simulink model "ProgettoControlli2_Simulink"  (R2025b)
settings: Solver=VariableStepAuto  StartTime=0.0  StopTime=240  RelTol=1e-3
values from neighbouring files (symbols this model uses):
  beta = 0.08    [progetto.m]    (also in progetto_alternativo.m)
  c = 6.2    [progetto.m]    (also in progetto_alternativo.m)
  Cth = 25.1 * 10^(-3)    (= 0.0251)    [progetto.m]    (also in progetto_alternativo.m)
  dlmax = l/100 * 4    (= 0.006)    [progetto.m]    (also in progetto_alternativo.m)
  g = 9.80665    [progetto.m]    (also in progetto_alternativo.m)
  h = 6.55    [progetto.m]    (also in progetto_alternativo.m)
  J = 2 * 10^(-4)    (= 0.0002)    [progetto.m]    (also in progetto_alternativo.m)
  K_max = 3.92 * 10^3    (= 3920)    [progetto.m]    (also in progetto_alternativo.m)
  m = 0.04    [progetto.m]    (also in progetto_alternativo.m)
  r1 = 0.0045    [progetto.m]    (also in progetto_alternativo.m)
  r2 = 0.045    [progetto.m]    (also in progetto_alternativo.m)
  Re = 4.8    [progetto.m]    (also in progetto_alternativo.m)
  Rth = 16.7    [progetto.m]    (also in progetto_alternativo.m)
  S = pi*d*l    (= 9.42477796077e-05)    [progetto.m]    (also in progetto_alternativo.m)
  Tamb = celsiusToKelvin(24)    [progetto.m]    (also in progetto_alternativo.m)
  Tavg = celsiusToKelvin(70)    [progetto.m]    (also in progetto_alternativo.m)
  Tdiff = 20    [progetto.m]    (also in progetto_alternativo.m)
  Tp = celsiusToKelvin(15)    [progetto.m]    (also in progetto_alternativo.m)
settings Model: Creator=nic  LastModifiedBy=nic

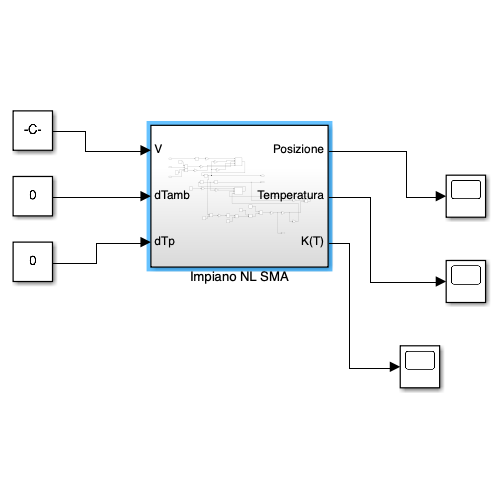
[thumbnail: Simulink's stored preview of the top-level diagram]
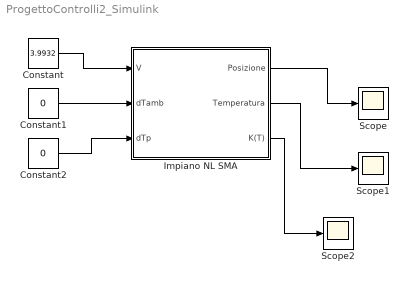
== system ProgettoControlli2_Simulink ==
  Constant : Constant  Value=3.9932
  Constant1 : Constant  Value=0
  Constant2 : Constant  Value=0
  Impiano NL SMA : Subsystem
  Scope : Scope
      settings: ActiveDisplayYMinimum=-57.097399679536004  ActiveDisplayYMaximum=15.047916213844935
  Scope1 : Scope
      settings: ActiveDisplayYMinimum=-115.33888478677272  ActiveDisplayYMaximum=597.203568929235
  Scope2 : Scope
      settings: ActiveDisplayYMinimum=-380.56361651334828  ActiveDisplayYMaximum=2443.7069252527017  DataLoggingVariableName=ScopeData2
  wires:
  Constant/1 -> Impiano NL SMA/1(V)
  Constant1/1 -> Impiano NL SMA/2(dTamb)
  Constant2/1 -> Impiano NL SMA/3(dTp)
  Impiano NL SMA/1(Posizione) -> Scope/1
  Impiano NL SMA/2(Temperatura) -> Scope1/1
  Impiano NL SMA/3(K(T)) -> Scope2/1

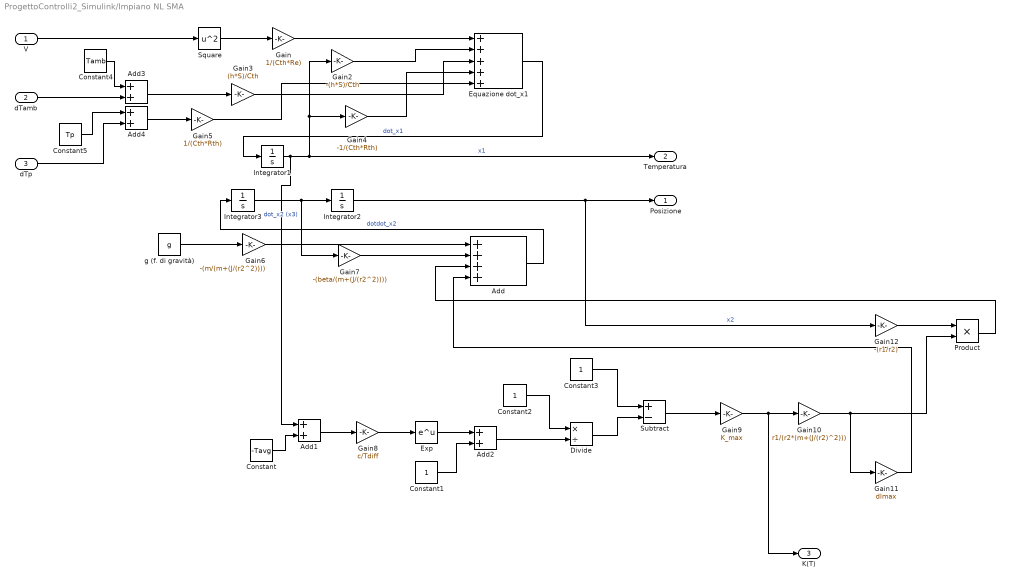
== system ProgettoControlli2_Simulink/Impiano NL SMA ==
  V : Inport
  dTamb : Inport  Port=2
  dTp : Inport  Port=3
  Add : Sum  Inputs=++++
  Add{1..4} (4 alike) : Sum
  Constant : Constant  Value=-Tavg
  Constant1 : Constant
  Constant2 : Constant
  Constant3 : Constant
  Constant4 : Constant  Value=Tamb
  Constant5 : Constant  Value=Tp
  Divide : Product  Inputs=*/
  Equazione dot_x1 : Sum  Inputs=+++++
  Exp : Math
  Gain : Gain  Gain=1/(Cth*Re)
  Gain10 : Gain  Gain=r1/(r2*(m+(J/(r2)^2)))
  Gain11 : Gain  Gain=dlmax
  Gain12 : Gain  Gain=-(r1/r2)
  Gain2 : Gain  Gain=-(h*S)/Cth
  Gain3 : Gain  Gain=(h*S)/Cth
  Gain4 : Gain  Gain=-1/(Cth*Rth)
  Gain5 : Gain  Gain=1/(Cth*Rth)
  Gain6 : Gain  Gain=-(m/(m+(J/(r2^2))))
  Gain7 : Gain  Gain=-(beta/(m+(J/(r2^2))))
  Gain8 : Gain  Gain=c/Tdiff
  Gain9 : Gain  Gain=K_max
  Integrator1 : Integrator
  Integrator2 : Integrator
  Integrator3 : Integrator
  Product : Product
  Square : Math  Operator=square
  Subtract : Sum  Inputs=+-
  g (f. di gravità) : Constant  Value=g
  Posizione : Outport
  Temperatura : Outport  Port=2
  K(T) : Outport  Port=3
  wires:
  V/1 -> Square/1
  Add/1 -> Integrator3/1  "dotdot_x2"
  Square/1 -> Gain/1
  Integrator2/1 -> Gain12/1, Posizione/1  "x2"
  Exp/1 -> Add2/1
  Gain7/1 -> Add/2
  g (f. di gravità)/1 -> Gain6/1
  Gain11/1 -> Add/4
  Constant3/1 -> Subtract/1
  Gain/1 -> Equazione dot_x1/1
  Add1/1 -> Gain8/1
  Add2/1 -> Divide/2
  Gain9/1 -> K(T)/1, Gain10/1
  Integrator3/1 -> Gain7/1, Integrator2/1  "dot_x2 (x3)"
  Gain10/1 -> Gain11/1, Product/2
  Divide/1 -> Subtract/2
  Constant2/1 -> Divide/1
  Gain3/1 -> Equazione dot_x1/3
  Gain6/1 -> Add/1
  Constant/1 -> Add1/2
  Gain5/1 -> Equazione dot_x1/5
  Gain8/1 -> Exp/1
  Subtract/1 -> Gain9/1
  Gain2/1 -> Equazione dot_x1/2
  Integrator1/1 -> Add1/1, Temperatura/1, Gain4/1, Gain2/1  "x1"
  Gain12/1 -> Product/1
  Constant1/1 -> Add2/2
  Gain4/1 -> Equazione dot_x1/4
  Product/1 -> Add/3
  Equazione dot_x1/1 -> Integrator1/1  "dot_x1"
  dTamb/1 -> Add3/2
  Constant4/1 -> Add3/1
  Add3/1 -> Gain3/1
  Constant5/1 -> Add4/1
  Add4/1 -> Gain5/1
  dTp/1 -> Add4/2
